simulink model "adamsFamillyModel"  (R2014b)
settings: Solver=ode45  StartTime=0.0  StopTime=wSimulationTime  FixedStep=T  MaxStep=wMaxStep  RelTol=1e-3
StopFcn:
  | save(wSaveFileName,wSaveFileName)
values from neighbouring files (symbols this model uses):
  wContinuousSystemDen = [1,11,30,200]    [AdamBashforthTutsin.m]    (also in AdamsBashforth.m; AdamsFamilly.m)
  wContinuousSystemNum = [100,0]    [AdamBashforthTutsin.m]    (also in AdamsBashforth.m; AdamsFamilly.m)
undefined symbols (not defined in the file or in its folder): A, B, C, D
settings Model: Creator=Zangdaarr  LastModifiedBy=Zangdaarr

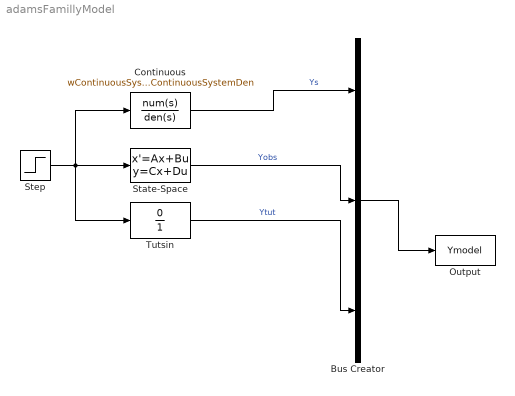
== system adamsFamillyModel ==
  Bus Creator : BusCreator  Inputs=3
  Continuous : TransferFcn  Numerator=wContinuousSystemNum  Denominator=wContinuousSystemDen
  Output : ToWorkspace  VariableName=Ymodel  SaveFormat=Timeseries  SampleTime=-1
  State-Space : StateSpace  A=A  B=B  C=C  D=D  X0=0
  Step : Step  Time=0  SampleTime=0
  Tutsin : DiscreteTransferFcn  Numerator=0  Denominator=[1]  SampleTime=0.1
  wires:
  Step/1 -> State-Space/1, Tutsin/1, Continuous/1
  Tutsin/1 -> Bus Creator/3  "Ytut"
  Bus Creator/1 -> Output/1
  State-Space/1 -> Bus Creator/2  "Yobs"
  Continuous/1 -> Bus Creator/1  "Ys"
